simulink model "model"  (R2022b)
settings: Solver=FixedStepAuto  StartTime=0.0  StopTime=20  FixedStep=0.001  RelTol=1e-3
undefined symbols (not defined in the file): A, A_M, b, b_M, gamma, P, theta
settings Model: Creator=Катя  LastModifiedBy=deniskirbaba
settings OptimizationCC: ReuseModelBlockBuffer=on

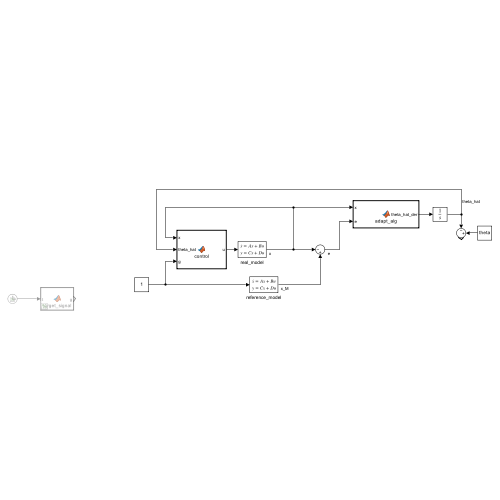
[thumbnail: Simulink's stored preview of the top-level diagram]
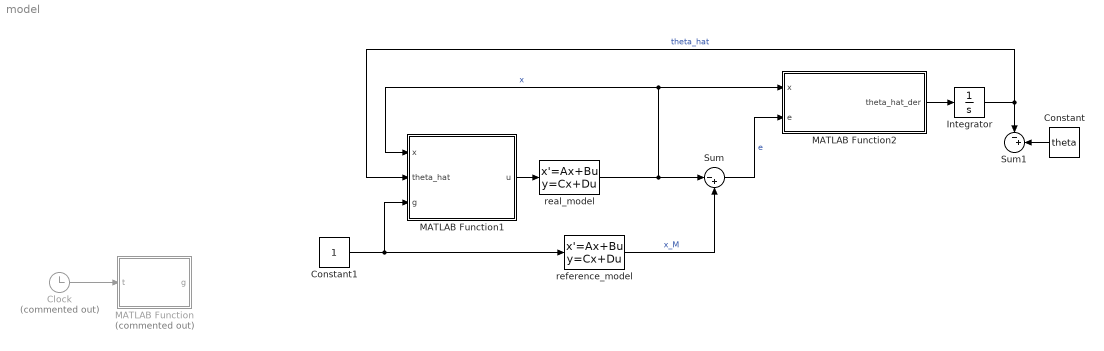
== system model ==
  Clock : Clock  Commented=on
  Constant : Constant  Value=theta
  Constant1 : Constant
  Integrator : Integrator
  MATLAB Function : MATLAB Function  Commented=on  TreatAsAtomicUnit=on
  MATLAB Function1 : MATLAB Function  TreatAsAtomicUnit=on
  MATLAB Function2 : MATLAB Function  TreatAsAtomicUnit=on
  Sum : Sum  Inputs=|-+
  Sum1 : Sum  Inputs=|-+
  real_model : StateSpace  A=A  B=b  C=eye(2)  D=[0; 0]  InitialCondition=[0; 0]
  reference_model : StateSpace  A=A_M  B=b_M  C=eye(2)  D=[0; 0]  InitialCondition=0
  wires:
  reference_model/1 -> Sum/2  "x_M"
  Clock/1 -> MATLAB Function/1(t)
  Constant1/1 -> MATLAB Function1/3(g), reference_model/1
  real_model/1 -> Sum/1, MATLAB Function2/1(x), MATLAB Function1/1(x)  "x"
  MATLAB Function1/1(u) -> real_model/1
  Sum/1 -> MATLAB Function2/2(e)  "e"
  MATLAB Function2/1(theta_hat_der) -> Integrator/1
  Integrator/1 -> MATLAB Function1/2(theta_hat), Sum1/1  "theta_hat"
  Constant/1 -> Sum1/2

== matlab function model/MATLAB Function1 ==
  data: x input; theta_hat input; u output; g input; kappa parameter
function u = control(x, theta_hat, g, kappa)
    u = theta_hat.' * x + g / kappa;
end

== matlab function model/MATLAB Function ==
  data: t input; g output
function g = target_signal(t)
    g = 7 * sign(cos(0.9 * t)) + 8;
end

== matlab function model/MATLAB Function2 ==
  data: x input; theta_hat_der output; e input; gamma parameter; b parameter; P parameter
function theta_hat_der = adapt_alg(x, e, gamma, b, P)
    theta_hat_der = gamma * x * b.' * P * e;
end
